simulink model "CRL_MCLV_V2_33EP256MC506_SlidingModeObserver_DualShunt_R2015a"  (R2015a)
settings: Solver=FixedStepDiscrete  StartTime=0.0  StopTime=10.0  FixedStep=.00005  RelTol=1e-3
PreLoadFcn:
  | UserParams;
values from neighbouring files (symbols this model uses):
  DELTA_STARTUP_RAMP = round( (MINSPEEDINRPM*POLEPAIRS*LOOPTIMEINSEC*LOOPTIMEINSEC*65536*65536/(60*OPENLOOPTIMEINSEC)) )    [UserParams.m]
  TS = LOOPTIMEINSEC    (= 5e-05)    [UserParams.m]
undefined symbols (not defined in the file or in its folder): A4, B15, B9, C5, C6, D8, F0, F1, Max, ms, P20, P41, P47, P53, P54, P96, P97, Pin, PWMmax, Resol, us
libraries: MCHP_Blockset x18, simulink x12
(part 1 of 2)
settings Model: Creator=M91449  LastModifiedBy=Lubin Kerhuel
settings DataIOCC: SaveFormat=Dataset
settings OptimizationCC: InlineParams=on  InlineInvariantSignals=on  OptimizeModelRefInitCode=on  LifeSpan=1
settings HardwareCC: ProdBitPerInt=16  ProdBitPerPointer=16  ProdLargestAtomicInteger=Integer  ProdIntDivRoundTo=Zero  ProdEndianess=LittleEndian  ProdWordSize=16  ProdHWDeviceType=Generic->Custom
settings ModelReferenceCC: ModelReferenceNumInstancesAllowed=Single
settings RTWCC: SystemTargetFile=MCHP_dsPIC_stf.tlc  TemplateMakefile=MCHP_dsPIC.tmf  Description=Microchip Embedded Target PIC24 dsPIC30 dsPIC33 (real-time)  GenerateReport=on  IncludeHyperlinkInReport=on  LaunchReport=on  GenerateTraceInfo=on  GenerateTraceReport=on  GenerateTraceReportSl=on  GenerateTraceReportSf=on  GenerateTraceReportEml=on  GenerateWebview=on  GenerateCodeMetricsReport=on  GenerateCodeReplacementReport=on
settings CodeAppCC: IgnoreCustomStorageClasses=off  MaxIdLength=255
settings STFCustomTargetCC: TargetLibSuffix=_lib.a  CodeReplacementLibrary=Microchip Code Replacement Library for dsPIC  GenerateSampleERTMain=off  IncludeMdlTerminateFcn=off  CombineOutputUpdateFcns=on  SuppressErrorStatus=on  SupportContinuousTime=off  SupportNonInlinedSFcns=on  SupportVariableSizeSignals=off  SystemTargetFile=MCHP_dsPIC_stf.tlc
settings ERTTargetCC: TargetLibSuffix=_lib.a  CodeReplacementLibrary=Microchip Code Replacement Library for dsPIC  GenerateSampleERTMain=off  IncludeMdlTerminateFcn=off  SuppressErrorStatus=on  SupportContinuousTime=off  SupportNonInlinedSFcns=on  SupportVariableSizeSignals=off  ERTSrcFileBannerTemplate=MCHP_dsPIC_code_template.cgt  ERTHdrFileBannerTemplate=MCHP_dsPIC_code_template.cgt  ERTDataSrcFileTemplate=MCHP_dsPIC_code_template.cgt  ERTDataHdrFileTemplate=MCHP_dsPIC_code_template.cgt  ERTCustomFileTemplate=MCHP_main.tlc

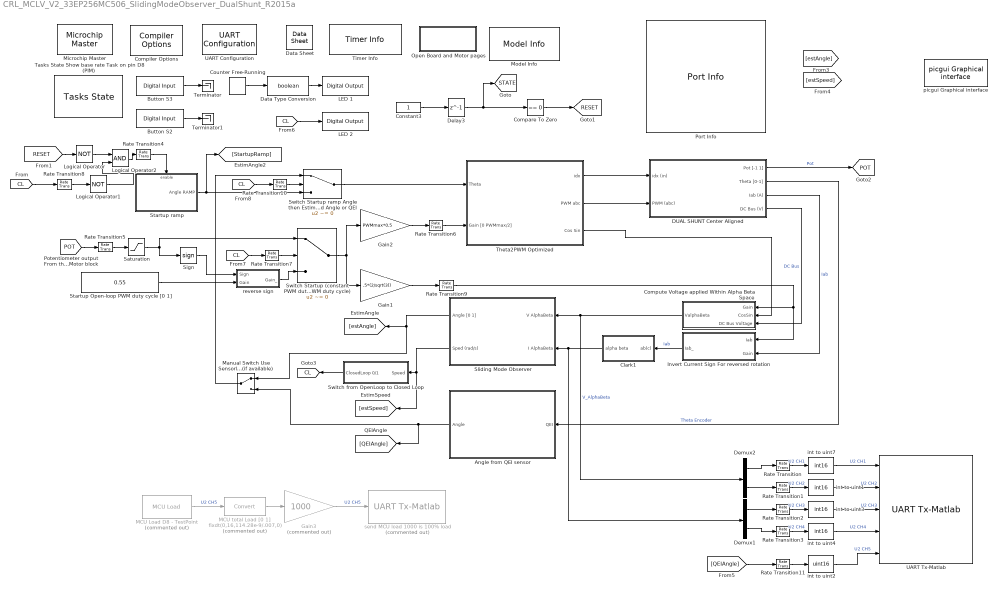
== system CRL_MCLV_V2_33EP256MC506_SlidingModeObserver_DualShunt_R2015a ==
  Angle from QEI sensor : Subsystem
  Button S2 : MCHP_Blockset/Digital IO/Digital Input  PORT=Dynamic Options  PORT_TXT="G   [ 6 : 9 ]"  PIN=7  PACK=off  SIMULTANEOUS=off  ORDERING=None  SampleTime=.1  MCHP_PORT={Digital In}{DIN}2:0:G7;  MCHP_MASTERLINK=CRL_MCLV_V2_33EP256MC506_SlidingModeObserver_DualShunt_R2015a/Microchip Master
  Button S3 : MCHP_Blockset/Digital IO/Digital Input  PORT=Dynamic Options  PORT_TXT="G   [ 6 : 9 ]"  PIN=6  PACK=off  SIMULTANEOUS=off  ORDERING=None  SampleTime=.1  MCHP_PORT={Digital In}{DIN}2:0:G6;  MCHP_MASTERLINK=CRL_MCLV_V2_33EP256MC506_SlidingModeObserver_DualShunt_R2015a/Microchip Master
  Clark1 : Subsystem
  Compare To Zero : simulink/Logic and Bit Operations/Compare To Zero  relop===  OutDataTypeStr=boolean
  Compiler Options : MCHP_Blockset/System Configuration/Compiler Options  Priority=1  LATEST_CMPLR=on  COMP_LIST=Dynamic Options  COMP_LIST_TXT=xc16 - v1.35  USE_64BIT_DOUBLE=off  MCHP_MULTITHREAD_COMPILATION=on  UseCustom_LinkerScript=off  MCHP_MASTERLINK=CRL_MCLV_V2_33EP256MC506_SlidingModeObserver_DualShunt_R2015a/Microchip Master  OPTIMIZATION_LEVEL=3  MPLAB_LINKLIB=default  MPLAB_LINKLIB1=default  UNROLL_LOOPS=on  OMIT_FRAME_POINTER=off  PROCEDURAL_ABSTRACTION=off  MCONST=in data memory  MDATA=Use only memory below address 8192 (faster)  MSCALAR=Use only memory below address 8192 (faster)  MCODE=is less than 32768 (faster)  HEAP_SIZE=0  OMF=elf  DEBUG_INFO=off  AssemblyListing=off  ProduceHexOutput=on
  Compute Voltage applied Within Alpha Beta Space : Subsystem
  Constant3 : Constant  OutDataTypeStr=uint16  SampleTime=.1
  Counter Free-Running : simulink/Sources/Counter Free-Running  NumBits=1  tsamp=.1
  DUAL SHUNT Center Aligned : Subsystem  VariantControl=(default)
  Data Sheet : MCHP_Blockset/System Info/Data Sheet  DOC_Type=datasheet  DOC_MCHP_Id=33EP256MC506_datasheet  DOC_FilePath=C:\Users\M91449\AppData\Local\Temp\70000657H.pdf  DOC_FileLastCheckTime="[2016              1             28             13             25         44.133]"  cpy_MCHP_Id=33EP256MC506  MCHP_MASTERLINK=CRL_MCLV_V2_33EP256MC506_SlidingModeObserver_DualShunt_R2015a/Microchip Master
      settings: AttributesFormatString=%<cpy_MCHP_Id>
  Data Type Conversion : DataTypeConversion  OutDataTypeStr=boolean
  Delay3 : Delay  DelayLength=1  InitialCondition=0
  Demux1 : Demux  Outputs=2
  Demux2 : Demux  Outputs=2
  Gain1 : Gain  Gain=.5*(2/sqrt(3))  OutDataTypeStr=fixdt(1,16,15)
  Gain2 : Gain  Gain=PWMmax*0.5  OutMin=-PWMmax*0.5  OutMax=PWMmax*0.5  OutDataTypeStr=fixdt(1,16)
  Gain3 : Gain  Commented=on  Gain=1000  OutDataTypeStr=uint16
  Invert Current Sign For reversed rotation : Subsystem
  LED 1 : MCHP_Blockset/Digital IO/Digital Output  PORT=Dynamic Options  PORT_TXT="D   [ 5  6  8 ]"  PIN=6  PACK=off  SIMULTANEOUS=off  READPREVIOUS=off  ORDERING=None  SampleTime=-1  MCHP_MASTERLINK=CRL_MCLV_V2_33EP256MC506_SlidingModeObserver_DualShunt_R2015a/Microchip Master
  LED 2 : MCHP_Blockset/Digital IO/Digital Output  PORT=Dynamic Options  PORT_TXT="D   [ 5  6  8 ]"  PIN=5  PACK=off  SIMULTANEOUS=off  READPREVIOUS=off  ORDERING=None  SampleTime=-1  MCHP_MASTERLINK=CRL_MCLV_V2_33EP256MC506_SlidingModeObserver_DualShunt_R2015a/Microchip Master
  Logical Operator : Logic  Operator=NOT  AllPortsSameDT=off  OutDataTypeStr=boolean
  Logical Operator1 : Logic  Operator=NOT  AllPortsSameDT=off  OutDataTypeStr=boolean
  Logical Operator2 : Logic  AllPortsSameDT=off  OutDataTypeStr=boolean
  MCU Load D8 - TestPoint : MCHP_Blockset/Profiling/MCU Load  Commented=on  MCULoadPin=Dynamic Options  MCULoadPin_TXT=None  MCULoadMeasure=on  TIMER_Resolution=Dynamic Options  TIMER_Resolution_TXT="Resol: 0.1143(us)  -  Max: 7.49(ms)"  MCHP_TIMER_REQUEST={MCU_Load}{MCU_Load}21:5:0:0:[]:524288;  MCHP_TIMER_RESULT=[1 65535 ]  MCHP_MASTERLINK=CRL_MCLV_V2_33EP256MC506_SlidingModeObserver_DualShunt_R2015a/Microchip Master  MCHP_COMPILED_INFO="CompiledSampleTime= [0.0070000000000000001   0 ];CompiledInportDataTypes=[ ];CompiledInportDataWidth=[];"  Info="Timer 1:  Resol: 114.2857143(ns)  -  Max: 7.48983(ms)"  SampleTime=.007
  MCU total Load [0 1] : DataTypeConversion  Commented=on  OutDataTypeStr=fixdt(0,16,114.28e-9/.007,0)  ConvertRealWorld=Stored Integer (SI)
  Manual Switch Use Sensorless Estimation or QEI (if available) : ManualSwitch
  Microchip Master : MCHP_Blockset/System Configuration/Microchip Master  Priority=1  PICREF=33EP256MC506  TIMESTEP_REF=ADC  BUSYFLAG=Dynamic Options  BUSYFLAG_TXT=D8 / Pin[42]  PWRTEN=Not used  BOREN=Disable  BODENV=2.7V  BORV=Not used  FPWRT=128ms  DSBOREN=Enable ZPBOR during Deep Sleep Mode  DSLPBOR=Not used  MCLRE=Enabled  SMCLR=MCLR pin generates a normal system Reset  PMDL1WAY=Allow only one reconfiguration  RSTPRI=Device will obtain reset instruction from Primary flash  TEMP=Not used  SOSCSRC=Not used  SOSCSEL=Not used  IOL1WAY=Allow only one reconfiguration  ALTVREF=Not used  DISUVREG=Not used  DSSWEN=Not used  LPCFG=Not used  RTCBAT=Not used  VBTBOR=Not used  WUTSEL=Not used  POWERSAVE=off  FNOSC=Primary Oscillator (XT; HS; EC)  FPR=ECIO w/ PLL 16x  FOSFPR=HS3 w/PLL 16x  FOS=Primary Oscillator  FRANGE=High Range  OSCILLATOR_SELECT=Crystal / Ceramic resonator  OSCILLATOR_SELECT_spd=Crystal / Ceramic resonator  QUARTZ=8e6  QUARTZ_spd=8e6  POSCGAIN=2x gain setting  POSCBOOST=Boost the kick start of the oscillator  SOSCGAIN=2x gain setting  SOSCBOOST=Boost the kick start of the oscillator  ACTIV_PLL=on  ACTIV_PLL_spd=on  MIPS_DESIRED=70e6  MIPS_DESIRED_spd=70e6  FPLLMUL=Not used  FPLLIDIV=8x Divider  POSCFREQ=Not used  POSCMD=XT Crystal Oscillator Mode  POSCMOD=Primary Oscillator Disabled  MIPS=70 * 1e6  ACLKCON=Optimized for PWM resolution & ADC conversion speed  FPLLODIV=32x Divider  PLLKEN=Clock switch to PLL source will wait until the PLL lock signal is valid.  FCKSM=Both Clock switching and Fail-safe Clock Monitor are enabled  FCKSMEN=Sw Disabled; Mon Disabled  IESO=Start up with FRC; then switch  DSWDTPS=1:2^36  FWDTEN=Disable  FWDTWINSZ=Window size is 25%  FWPSA=1:512  FWPSA0=1:128  FWPSB=1:16  WDT=Disable  WDTPOST=1:32768  WDTPRE=1:128  WDTPS=1:32768  WINDIS=Watchdog Timer in Non-Window mode  WWDTEN=Non-Window mode  DSWDTEN=Enable DSWDT during Deep Sleep Mode  DSWDTOSC=Select LPRC as DSWDT Reference clock  FPBDIV=Not used  FSOSCEN=Enable SOSC  LPRCSEL=Not used  OSCIOFCN=Not used  OSCIOFNC=general purpose digital I/O pin  LVRCFG=Not used  PLL_96MHZ=Not used  PLL96MHZ=Not used  PLLDIV=Not used  WDTCLK=Not used  WDTCMX=Not used  WDTWIN=WDT Window is 25% of WDT period  APL=Aux Flash Code protect is disabled  APLK=Aux Flash Write Protection or Code Protection is Enabled  AWRP=Auxiliary program memory is not write-protected  BSS=No Boot program Flash segment  BWP=Not used  BWRP=Boot Segment may be written  CP=Protection Disabled  EBS=No Boot EEPROM  ESS=No Segment Data EEPROM  GCP=General Segment Code protect is Disabled  GSS=General Segment Code protect is Disabled  GSS0=Not used  GSSK=General Segment Write Protection or Code Protection is Enabled  GWRP=General Segment may be written  PWP=Not used  RBS=No Boot RAM  RSS=No Secure RAM  SSS=No Secure Segment  SWRP=Secure segment may be written  WPCFG=Not used  WPDIS=Not used  WPEND=Not used  WPFP=Not used  ICESEL=Communicate on PGEC1/PGED1  ICS=Communicate on PGEC2 and PGED2  JTAGEN=Disable  COE=Not used  RES=Not used  DEBUG=Debugger is disabled  BACKBUG=Not used  BKBUG=Not used  ALTI2C=I2C mapped to SDA1/SCL1 pins  ALTI2C1=I2C1 mapped to SDA1/SCL1 pins  ALTI2C2=I2C2 mapped to SDA2/SCL2 pins  ALTQIO=QEA1; QEB1; INDX1 are selected as inputs to QEI1  ALTSS1=SS1A is selected as the I/O pin for SPI1  CMPPOL0=Hysteresis is applied to falling edge  CMPPOL1=Hysteresis is applied to falling edge  FCANIO=Not used  FETHIO=Default Ethernet I/O  FMIIEN=MII Enabled  FSRSSEL=Not used  FUSBIDIO=Controlled by the USB Module  FVBUSONIO=Not used  HPOL=PWM module high side output pins have active-high output polarity  HYST0=45 mV Hysteresis  HYST1=45 mV Hysteresis  I2C1SEL=Not used  LPOL=PWM module low side output pins have active-high output polarity  PWMPIN=PWM module pins controlled by PORT register at device Reset  RTCOSC=Not used  UPLLEN=USB PLL Disabled  UPLLIDIV=Not used  ATMOD8=Not used  ALTPMP=Not used  I2C2SEL=Not used  ALTADREF=Not used  ALTCVREF=Not used  PWMLOCK=PWM registers may be written without key sequence  MCHP_TIMER_RESULT=[ ]  MCHP_PORT={Busy Flag}{Busy}0:1:D8;  MCHP_PLLRegisters="[5    243  16385     -1]"  MCHPVAR=MCHP.fcy.MIPS=70000000;MCHP.fcy.SYSCLK=70000000;MCHP.fcy.ADC=70000000;MCHP.fcy.Comparator=70000000;MCHP.fcy.I2C=70000000;MCHP.fcy.SPI=70000000;MCHP.fcy.UART=70000000;MCHP.fcy.Timers=70000000;MCHP.fcy.OC=70000000;MCHP.fcy.IC=70000000;MCHP.fcy.Ports=70000000;MCHP.fcy.QEI=70000000;MCHP.PowerSave=0;MCHP.TimeStepFactor=-20000;MCHP.TimeStep_Timer=-1;MCHP.NTIMERS=5;MCHP.id.name='33EP256MC506';MCHP.id.N=reshape([33 256 506],1,3);MCHP.id.L=reshape({ 'EP','MC',''},1,3);MCHP.id.Arch=3;MCHP.periph.PPS.reg_RPINRx=reshape([-1 1 1 -1 -1 -1 1 -1 -1 -1 -1 -1 -1 -1 1 1 1 1 -1 -1 -1 -1 -1 -1 1 1 -1 -1 1 1 1 1 -1 -1 -1 -1 1 -1 1 -1 -1 -1 -1 -1 1 1 1 -1 -1 -1 -1 -1 1 -1 -1 -1 -1 -1 -1 -1 -1 -1 -1 -1 -1 -1 -1 -1 -1 -1 -1 -1 -1 -1 -1 1 -1 1 1 1],1,80);MCHP.PPS.dsPIC.RP=reshape([-1 -1 -1 -1 -1 -1 -1 -1 -1 -1 -1 -1 -1 -1 -1 -1 -1 -1 -1 -1 4 -1 -1 -1 -1 -1 -1 -1 -1 -1 -1 -1 -1 -1 -1 19 20 21 22 23 24 25 26 27 -1 -1 -1 -1 -1 -1 -1 -1 -1 -1 38 39 40 41 -1 -1 -1 -1 -1 -1 -1 -1 -1 -1 -1 -1 -1 -1 -1 -1 -1 -1 -1 -1 -1 -1 -1 -1 -1 -1 -1 -1 -1 -1 -1 -1 -1 -1 -1 -1 -1 -1 -1 81 -1 -1 -1 -1 -1 -1 -1 -1 -1 -1 -1 -1 -1 -1 -1 -1 -1 -1 -1 -1 102 -1 104],1,121);MCHP.PPS.dsPIC.RPI=reshape([-1 -1 -1 -1 -1 -1 -1 -1 -1 -1 -1 -1 -1 -1 -1 -1 -1 -1 -1 -1 -1 -1 -1 -1 8 9 -1 11 12 -1 -1 -1 16 17 18 -1 -1 -1 -1 -1 -1 -1 -1 -1 28 29 30 31 -1 -1 -1 35 36 37 -1 -1 -1 -1 42 -1 -1 -1 -1 -1 -1 -1 -1 -1 -1 -1 -1 -1 -1 -1 -1 -1 -1 -1 -1 -1 -1 -1 -1 -1 -1 -1 -1 -1 -1 -1 -1 -1 -1 -1 78 79 80 -1 -1 -1 -1 -1 -1 -1 -1 -1 -1 -1 -1 -1 -1 -1 -1 -1 -1 -1 -1 -1 -1 103 -1 105],1,122);MCHP.PPS.dsPIC.RPINR_list=reshape({ '1','INT1','INT2','INT3','INT4','T1CK','T2CK','T3CK','T4CK','T5CK','T6CK','T7CK','T8CK','T9CK','IC1','IC2','IC3','IC4','IC5','IC6','IC7','IC8','OCFA','OCFB','FLT1','FLT2','FLT3','FLT4','QEA1','QEB1','INDX1','HOME1','QEA2','QEB2','INDX2','HOME2','U1RX','U1CTS','U2RX','U2CTS','SDI1','SCK1_in','SS1_in','44','SDI2','SCK2_in','SS2_in','48','CSDIR','CSCK','COFS','52','C1RX','C2RX','U3RX','U3CTS','U4RX','U4CTS','SDI3','SCK3_in','SS3_in','62','SDI4','SCK4_in','SS4_in','66','IC9','IC10','IC11','IC12','IC13','IC14','IC15','IC16','OCFC','SYNCI1','SYNCI2','DTCMP1','DTCMP2','DTCMP3','DTCMP4','DTCMP5','DTCMP6','DTCMP7','FLT5','FLT6','FLT7','FLT8','89','SENT1','SENT2','92'},1,92);MCHP.PPS.dsPIC.RPOR_list=reshape({ '1','U1TX','U1RTS','U2TX','U2RTS','SDO1','SCK1_out','SS1_out','SDO2','SCK2_out','SS2_out','CSDO','CSCK','COFS','C1TX','C2TX','OC1','OC2','OC3','OC4','OC5','OC6','OC7','OC8','C1OUT','C2OUT','C3OUT','U3TX','U3RTS','U4TX','U4RTS','SDO3','SCK3_out','SS3_out','SDO4','SCK4_out','SS4_out','OC9','OC10','OC11','OC12','OC13','OC14','OC15','OC16','SYNCO1','SYNCO2','QEI1CCMP','QEI2CCMP','REFCLK','C4OUT','C5OUT','52','53','54','55','56','SENT1','SENT2'},1,59);MCHP.PPS.map_RPnR_RPORx=reshape([20 35 36 37 38 39 40 41 42 43 54 55 56 57 -1 97 -1 118 120],1,19);MCHP.Rx=reshape([13 15 21 -1 -1 58 -1 -1 -1 -1 -1 14 16 22 -1 -1 59 -1 -1 -1 -1 -1 -1 17 23 -1 -1 -1 -1 -1 -1 -1 -1 -1 18 35 -1 -1 -1 -1 -1 -1 -1 -1 33 32 36 -1 -1 -1 -1 -1 -1 -1 -1 -1 43 37 53 -1 -1 -1 -1 -1 -1 -1 -1 44 50 54 -1 -1 4 -1 -1 -1 -1 1 46 51 -1 -1 -1 5 -1 -1 -1 -1 31 48 52 42 -1 -1 6 -1 -1 -1 -1 34 49 55 -1 -1 -1 8 -1 -1 -1 -1 64 60 45 -1 -1 -1 -1 -1 -1 -1 -1 12 61 24 -1 -1 -1 -1 -1 -1 -1 -1 11 62 39 -1 27 -1 -1 -1 -1 -1 -1 -1 63 47 -1 28 -1 -1 -1 -1 -1 -1 -1 2 -1 -1 29 -1 -1 -1 -1 -1 -1 -1 3 40 -1 30 -1 -1 -1 -1 -1 -1],11,16);MCHP.ADC.ANtype=reshape([3 0],1,2);MCHP.ADC.ADCONx=reshape([47103 59391 40959 263 0 0],1,6);MCHP.ADC.ADCHS_0=reshape([40863 1799],1,2);MCHP.ADC.Flags=reshape([1 0],1,2);MCHP.ADC.Buffer=reshape([16 -1],1,2);MCHP.ADC.port=reshape([0 1 16 17 18 19 32 33 34 11 12 43 76 77 78 79 -1 -1 -1 -1 -1 -1 -1 -1 -1 -1 -1 -1 -1 -1 -1 -1 -1 -1 -1 -1 -1 -1 -1 -1 -1 -1 -1 -1 -1 -1 -1 -1 -1 -1 -1 -1 -1 -1 -1 -1 -1],1,57);MCHP.ADC.port_ALT=reshape([-1 -1 -1 -1],1,4);MCHP.ADC.port_VrefP=17;MCHP.ADC.port_VrefM=16;MCHP.ADC.port_AVdd=-1;MCHP.ADC.port_AVss=-1;MCHP.ADC.ADCDATA=reshape([0 0 0 0 0 0 0 0 0 0 0 0 0 0 0 0 0 0 0 0 0 0 0 0 0 0 0 0 0 0 0 0 0 0 0 0 0 0 0 0 0 0 0 0 0 0 0 0 0 0 0 0 0 0 0 0 0],1,57);MCHP.memory.RAM=32768;MCHP.memory.RAM_XBegin=4096;MCHP.memory.RAM_YBegin=20480;MCHP.memory.RAM_dma=reshape([-1 -1],1,2);MCHP.memory.FLASH_ECC=0;MCHP.DMA.Num=4;MCHP.DMA.CNTmax=16383;MCHP.QEI.QEICONx=reshape([49023 -1 -1 -1 -1 -1],1,6);MCHP.QEI.QEItype=1;MCHP.QEI.Port_QEI_INDX=reshape([-1 -1],1,2);MCHP.QEI.Port_QEI_QEA=reshape([-1 -1],1,2);MCHP.QEI.Port_QEI_QEB=reshape([-1 -1],1,2);MCHP.QEI.Port_QEI_UPDN=reshape([-1 -1],1,2);MCHP.INT.Port=reshape([23 32767 32767 -1 -1],1,5);MCHP.PWM_HS.Flags=reshape([3 1 0],1,3);MCHP.PWM.port_FLT=reshape([-1 -1 -1 34 43 -1 -1 -1 -1 -1 -1 -1 -1 -1 -1 -1 -1 -1 -1 -1 -1 -1 -1 -1 -1 -1 -1 -1 -1 -1 -1 -1 20],1,33);MCHP.PWM.PWMRef=-1;MCHP.PWM.Flag=0;MCHP.PWM.Port_PWM_l=reshape([31 -1 29 -1 27 -1 -1 -1 -1 -1 -1 -1 -1 -1 -1 -1 -1 -1 -1 -1 -1 -1 -1 -1],2,12);MCHP.PWM.Port_PWM_h=reshape([30 -1 28 -1 26 -1 -1 -1 -1 -1 -1 -1 -1 -1 -1 -1 -1 -1 -1 -1 -1 -1 -1 -1],2,12);MCHP.IC.Port=reshape([32767 32767 32767 32767 0 0 0 0 0 0 0 0 0 0 0 0],1,16);MCHP.IC.type=1;MCHP.OC.Port=reshape([32767 32767 32767 32767 0 0 0 0 0 0 0 0 0 0 0 0],1,16);MCHP.OC.type=1;MCHP.CN.Port=reshape([-1 -1 -1 -1 -1 -1 -1 -1 -1 -1 -1 -1 -1 -1 -1 -1 -1 -1 -1 -1 -1 -1 -1 -1 -1 -1 -1 -1 -1 -1 -1 -1 -1 -1 -1 -1 -1 -1 -1 -1 -1 -1 -1 -1 -1 -1 -1 -1 -1 -1 -1 -1 -1 -1 -1 -1 -1 -1 -1 -1 -1 -1 -1 -1 -1 -1 -1 -1 -1 -1 -1 -1 -1 -1 -1 -1 -1 -1 -1 -1 -1 -1 -1 -1 -1],1,85);MCHP.CN.PullUp=reshape([8083 65535 49151 352 61440 3 960 0 0 0 0],1,11);MCHP.CN.type=1;MCHP.CN.Flag_PullDown=1;MCHP.SPI.Refs=reshape([1 2 0 0 0 0],1,6);MCHP.SPI.SPIxCON1=8191;MCHP.SPI.SPIxCON2=57347;MCHP.SPI.Port_SDI=reshape([9 -1 -1 -1 -1 -1],1,6);MCHP.SPI.Port_SDO=reshape([4 -1 -1 -1 -1 -1],1,6);MCHP.SPI.Port_SCK=reshape([35 -1 -1 -1 -1 -1],1,6);MCHP.SPI.Port_SS=reshape([16 -1 -1 -1 -1 -1],1,6);MCHP.I2C.Refs=reshape([1 2 0 0 0],1,5);MCHP.I2C.I2CxCON=49151;MCHP.I2C.NewRegName=1;MCHP.I2C.Port_SDA=reshape([36 8 -1 -1 -1],1,5);MCHP.I2C.Port_SCL=reshape([37 20 -1 -1 -1],1,5);MCHP.I2C.Port_ASDA=reshape([25 21 -1 -1 -1],1,5);MCHP.I2C.Port_ASCL=reshape([24 22 -1 -1 -1],1,5);MCHP.I2C.Fuse_Port_SCL_SDA=reshape([3 1 4 1 -1 -1 -1 -1 -1 -1],2,5);MCHP.I2C.Fuse_Port_ASCL_ASDA=reshape([3 2 4 2 -1 -1 -1 -1 -1 -1],2,5);MCHP.PGA.Port_PGA1P=reshape([-1 -1 -1 -1],1,4);MCHP.PGA.Port_PGA1N=reshape([-1 -1 -1 -1],1,4);MCHP.PGA.Port_PGA2P=reshape([-1 -1 -1 -1],1,4);MCHP.PGA.Port_PGA2N=reshape([-1 -1 -1 -1],1,4);MCHP.PGA.Num=0;MCHP.HS_AnalogComparator.Port_CMP1=reshape([-1 -1 -1 -1],1,4);MCHP.HS_AnalogComparator.Port_CMP2=reshape([-1 -1 -1 -1],1,4);MCHP.HS_AnalogComparator.Port_CMP3=reshape([-1 -1 -1 -1],1,4);MCHP.HS_AnalogComparator.Port_CMP4=reshape([-1 -1 -1 -1],1,4);MCHP.HS_AnalogComparator.PORT_EXTREFx=reshape([-1 -1],1,2);MCHP.HS_AnalogComparator.Port_DACOUTx=reshape([-1 -1],1,2);MCHP.HS_AnalogComparator.Num=0;MCHP.Comp.Port_CVrefin=-1;MCHP.Comp.Port_CVref=-1;MCHP.Comp.Port_CVref1O=24;MCHP.Comp.Port_CVref2O=4;MCHP.Comp.Port_CxOUT=reshape([32767 32767 32767 32767 -1],1,5);MCHP.Comp.Port_OAxOUT=reshape([17 0 32 -1 -1],1,5);MCHP.Comp.Port_CxINP=reshape([18 1 34 32 -1],1,5);MCHP.Comp.Port_CxINM=reshape([19 43 -1 -1 16 76 -1 -1 33 77 -1 -1 33 -1 -1 -1 -1 -1 -1 -1],4,5);MCHP.Comp.nComp=reshape([4 0 0],1,3);MCHP.Comp.OpAmp=7;MCHP.Comp.CVRCON=reshape([17663 0],1,2);MCHP.CDAC.Port_DACx=reshape([-1 -1 -1],1,3);MCHP.CDAC.nCDAC=0;MCHP.UART.port_Rx=reshape([32767 32767 -1 -1 -1 -1],1,6);MCHP.UART.port_Tx=reshape([32767 32767 -1 -1 -1 -1],1,6);MCHP.UART.port_ARx=reshape([-1 -1],1,2);MCHP.UART.port_ATx=reshape([-1 -1],1,2);MCHP.UART.port_RTS=reshape([34 76 -1 -1 -1 -1],1,6);MCHP.UART.port_CTS=reshape([43 77 -1 -1 -1 -1],1,6);MCHP.UART.reg_UxMODE=reshape([48127 48127 -1 -1 -1 -1],1,6);MCHP.UART.reg_UxSTA=reshape([61439 61439 -1 -1 -1 -1],1,6);MCHP.modsrc.DOS_00794=1;MCHP.modsrc.DOS_00931=1;MCHP.modsrc.DOS_00932=1;MCHP.modsrc.DOS_00942=1;MCHP.modsrc.DOS_00938=1;MCHP.modsrc.DOS_00996=1;MCHP.modsrc.DOS_00997=1;MCHP.modsrc.DOS_00998=1;MCHP.modsrc.DOS_00209=0;MCHP.modsrc.DOS_01555_adc=0;MCHP.modsrc.DOS_01293=1;MCHP.modsrc.DOS_00828=0;MCHP.modsrc.DOS_01116=1;MCHP.modsrc.DOS_01017_RPORx=1;MCHP.modsrc.DOS_01017_RPINRx=1;MCHP.modsrc.DOS_01555_nvm_tsmc18_v2_16bit=0;MCHP.modsrc.DOS_00804=1;MCHP.modsrc.DOS_00826=1;MCHP.modsrc.DOS_01555_TLAK_PMDx=0;MCHP.modsrc.DOS_01555_TLAK_INT_=0;MCHP.modsrc.DOS_00933=1;MCHP.modsrc.DOS_01555=0;MCHP.modsrc.DOS_01555_ptg=0;MCHP.modsrc.DOS_00929=1;MCHP.modsrc.DOS_00958=1;MCHP.modsrc.DOS_01117_PORTx=1;MCHP.modsrc.DOS_00999=0;MCHP.modsrc.DOS_01198=1;MCHP.modsrc.DOS_01041=1;MCHP.modsrc.DOS_00892=1;MCHP.modsrc.DOS_01287_TLAC_PMDx=1;MCHP.modsrc.DOS_01287_TLAC_INT_=1;MCHP.modsrc.DOS_01424=1;MCHP.modsrc.DOS_01332=1;MCHP.modsrc.DOS_01441_i2c_upb_v1_16bit_TLAH=0;MCHP.modsrc.DOS_01482=0;MCHP.modsrc.DOS_02508c11=0;MCHP.modsrc.DOS_01468_PMBA_current_source=0;MCHP.modsrc.DOS_02291_PGA=0;MCHP.modsrc.DOS_01467_Comparator=0;MCHP.modsrc.DOS_01498_TLAY=0;MCHP.modsrc.DOS_02316_nvm_ctrl_v1_16bit=0;MCHP.modsrc.DOS_00993_PLL_120MHz=0;MCHP.modsrc.DOS_01577_cla_clc_upb_v1=0;MCHP.modsrc.DOS_01332_ptg_pc_v1=0;MCHP.modsrc.DOS_00958_pwm_TLAY=0;MCHP.modsrc.TLAY_IOPorts=0;MCHP.modsrc.DOS_00929q=0;MCHP.modsrc.DOS_02415_spi_v5=0;MCHP.modsrc.DOS_RPINRx_16bit_2=0;MCHP.modsrc.DOS_01497_TLAH_PMDx=0;MCHP.modsrc.DOS_02550_TLAL_INT=0;MCHP.modsrc.DOS_00958_pwm_TLAH=0;MCHP.modsrc.DOS_01287_TLAH_INT_=0;MCHP.modsrc.DOS_01113=0;MCHP.modsrc.DOS_01017_PMDx=0;MCHP.modsrc.DOS_00927=0;MCHP.modsrc.DOS_01080=0;MCHP.modsrc.DOS_00794_cpu_16bit_v3=0;MCHP.modsrc.DOS_02359a_sent_j2716_upb_v1=0;MCHP.modsrc.DOS_01520_wdt_dmt_upb_v1_16bit=0;MCHP.modsrc.DOS_02192_TLCD_PMDx=0;MCHP.modsrc.DOS_02192_TLCD_INT_=0;MCHP.modsrc.DOS_02192_cmp=0;MCHP.modsrc.DOS_00958_pwm_TLCD=0;MCHP.modsrc.DOS_02192_PORTx_TLCD=0;MCHP.modsrc.DOS_00936=0;MCHP.modsrc.DOS_00995=0;MCHP.modsrc.DOS_00546=0;MCHP.modsrc.DOS_00474=0;MCHP.modsrc.DOS_02481_WACJ_Config=0;MCHP.modsrc.DOS_02569_pfm_cache_ocp_v1=0;MCHP.modsrc.DOS_02819_pfm_ctrl_32bit_upb_v2=0;MCHP.modsrc.DOS_02674_wdt_upb_v1_32bit=0;MCHP.modsrc.DOS_01520_wdt_dmt_upb_v1=0;MCHP.modsrc.DOS_02869_icd_jtag_bvci_upb_v2=0;MCHP.modsrc.DOS_02823_WACJ_clk_cru_upb_v2=0;MCHP.modsrc.DOS_01423_RPINRx=0;MCHP.modsrc.DOS_02481_RPORx=0;MCHP.modsrc.DOS_02511_pwr_sib_upb_v1_32bit=0;MCHP.modsrc.DOS_02481_WACJ_int_evic_v3=0;MCHP.modsrc.DOS_01500_dma_bvci_v2=0;MCHP.modsrc.DOS_02141_tmr_classa_pb_v2=0;MCHP.modsrc.DOS_02815_tmr_classb_upb_v1=0;MCHP.modsrc.DOS_00740_icap_pb_v1=0;MCHP.modsrc.DOS_00749_ocmp_pb_v1=0;MCHP.modsrc.DOS_01441_i2c_upb_v1_32bit=0;MCHP.modsrc.DOS_01329_spi_pb_v2=0;MCHP.modsrc.DOS_02478_uart_irda_upb_v1_32bit=0;MCHP.modsrc.DOS_02514_dfm_strl_sst_upb_v1=0;MCHP.modsrc.DOS_01427_cmp_control_upb_v1_32bit=0;MCHP.modsrc.DOS_01445_dac_nbit__control_upb_v1_32bit=0;MCHP.modsrc.DOS_01461_afe_ctmu_con_upb_v1=0;MCHP.modsrc.DOS_02472_ppi_pmp16_upb_v1=0;MCHP.modsrc.DOS_02467_gpio_ports_upb_v1=0;MCHP.modsrc.DOS_02508_adc_sar_ctrl_upb_v1_PIC32MK=0;MCHP.modsrc.DOS_02813a_usb_otgcore_pb_v3=0;MCHP.modsrc.DOS_01261_tmr_rtcc_pb_v2=0;MCHP.modsrc.DOS_01475_lpwr_deep_sleep_ctrl_v2=0;MCHP.modsrc.DOS_EIP_00136_ssx_v1=0;MCHP.modsrc.DOS_01152_can_bvci_v1=0;MCHP.modsrc.DOS_02481_WACN_Config=0;MCHP.modsrc.DOS_02823_WACN_clk_cru_upb_v2=0;MCHP.modsrc.DOS_02481_WACN_int_evic_v3=0;MCHP.modsrc.DOS_03554_cmp_control_upb_v2_32bit=0;MCHP.modsrc.DOS_01577_cla_clc_upb_v1_32bit=0;MCHP.modsrc.DOS_03247_can_fd_upb_v2=0;MCHP.modsrc.DOS_02481_WACK_MC_Config=0;MCHP.modsrc.DOS_03247_can_fd_upb_v2_pic32mk=0;MCHP.modsrc.DOS_02481_WACJ_MC_Config=0;MCHP.modsrc.DOS_02481_WACJ_MC_int_evic_v3=0;MCHP.modsrc.DOS_01477_pwm_mc_upb_v1=0;MCHP.modsrc.DOS_01459_ptg_pc_upb_v1_SIC=0;MCHP.modsrc.DOS_01494_qei_32b_upb_v1=0;MCHP.modsrc.DOS_02481_WACN_MC_Config=0;MCHP.modsrc.DOS_02481_WACN_MC_int_evic_v3=0;MCHP.modsrc.DOS_02787_WACD_Config=0;MCHP.modsrc.DOS_00800_dac_4bit_ctrl_pb_v1=0;MCHP.modsrc.DOS_01539_icd_jtag_pb_v2=0;MCHP.modsrc.DOS_02823_clk_cru_upb_v2=0;MCHP.modsrc.DOS_01423_RPORx=0;MCHP.modsrc.DOS_02907_WACD_int_evic_v3=0;MCHP.modsrc.DOS_00734_uart_irda_pb_v1=0;MCHP.modsrc.DOS_00687_tmr_classa_pb_v1=0;MCHP.modsrc.DOS_00745_tmr_classb_pb_v1=0;MCHP.modsrc.DOS_02508_adc_sar_ctrl_upb_v1=0;MCHP.modsrc.DOS_00866_cmp_control_pb_v2=0;MCHP.modsrc.DOS_01114_eth_bvci_v1=0;MCHP.modsrc.DOS_02831_usb_clk_rst_v2=0;MCHP.modsrc.DOS_01643_pfm_cache_ahb_v2=0;MCHP.modsrc.DOS_EIP_00206r5_sqi_v2=0;MCHP.modsrc.DOS_EIP_00124_usb_hs_otgcore_v1=0;MCHP.modsrc.DOS_EIP_00218_math_rng_ahbs_v2=0;MCHP.modsrc.DOS_EIP_00109_ebi_v1=0;MCHP.modsrc.DOS_EIP_00158_crypto_v1=0;MCHP.clock.PBxDIV=-1;  MCHP_CRC=5766771  BTMODE=Not used  RES1=Not used  PLLSS=Not used  RES2=Not used  ALTCMPI=Not used  BOREN1=Not used  ALTRB6=Not used  RETCFG=Not used  DFMCY=Not used  BSS2=No Boot Segment  BSEN=No Boot Segment  CWRP=Configuration Segment may be written  CSS=No Protection (other than CWRP)  AIVTDIS=Disable Alternate Vector Table  BSLIM=Not used  WDTEN=Disable  BTSWP=BOOTSWP instruction is disabled  DBCC=No Cross Connection between DAC outputs  CTXT1=Not Assigned  CTXT2=Not Assigned  SEQNUM=Not used  nSEQNUM=Not used  BOREN0=Enabled  DMTIVT=Not used  DMTCNT=2^31 (2147483648)  DMTEN=Dead Man Timer is Disabled and can be enabled by software  ON=Not used  USERID=Not used  RESERVED1=Not used  PGL1WAY=Allow only one reconfiguration  FPLLRNG=34-68 MHz Input  FPLLICLK=FRC is input to the System PLL  FPLLMULT=PLL Multiply by 128  UPLLFSEL=USB PLL input is 24 MHz  DMTINTV=Window/Interval value is 127/128 counter value  WDTSPGM=WDT stops during Flash programming  FDMTEN=Deadman Timer is disabled  TRCEN=Trace features in the CPU are enabled  BOOTISA=Boot code and Exception code is MIPS32  FECCCON=ECC and Dynamic ECC are disabled (ECCCON bits are writable)  EXTDDRSIZE=Not used  FSLEEP=Flash is powered down when the device is in Sleep mode  DBGPER=Allow CPU access to all permission regions  EJTAGBEN=Normal EJTAG functionality  TSEQ=Not used  CSEQ=Not used
  Model Info : simulink/Model-Wide Utilities/Model Info  Frame=on  DisplayStringWithTags=|  HorizontalTextAlignment=Left  LeftAlignmentValue=0.02  SourceBlockDiagram=CRL_MCLV_V2_33EP256MC506_SlidingModeObserver_DualShunt_R2015a  TagMaxNumber=20
      | Short hust motor with:
      | M1 - Black
      | M2 - Red
      | M3 - White
  Open Board and Motor pages : Subsystem
      settings: OpenFcn=|
      | web('www.microchip.com/DevelopmentTools/ProductDetails.aspx?PartNO=DM330021-2','-browser');
      | pause(1);
      | web('http://www.microchipdirect.com/productsearch.aspx?keywords=AC300020','-browser');
      | pause(1);
      | web('www.microchipdirect.com/ProductSearch.aspx?keywords=AC300022','-browser');
      mask Display: disp('Open tools\nWebpage');
  Port Info : MCHP_Blockset/System Info/Port Info  MCHP_MASTERLINK=CRL_MCLV_V2_33EP256MC506_SlidingModeObserver_DualShunt_R2015a/Microchip Master
  Rate Transition{,1..4,6..11} (11 alike) : RateTransition
  Rate Transition5 : RateTransition  OutPortSampleTime=.1
  Saturation : Saturate  UpperLimit=1  LowerLimit=0
  Sign : Signum
  Sliding Mode Observer : Subsystem
  Startup Open-loop PWM duty cycle [0 1] : Constant  Value=0.55  OutDataTypeStr=Inherit: Inherit via back propagation
  Startup ramp : Subsystem
  Switch Startup (constant PWM duty cycle) then Closed Loop (Pot drive PWM duty cycle) : Switch  Criteria=u2 ~= 0  Threshold=250
  Switch Startup ramp Angle then Estimated Angle or QEI : Switch  Criteria=u2 ~= 0  Threshold=250
  Switch from OpenLoop to Closed Loop : Subsystem
  Tasks State Show base rate Task on pin D8 (PIM) : MCHP_Blockset/Profiling/Tasks State  TasksPin=D8  MCHP_PORT={Task D1 Running}{Task D1}15:1:D8;  MCHP_MASTERLINK=CRL_MCLV_V2_33EP256MC506_SlidingModeObserver_DualShunt_R2015a/Microchip Master
  Terminator : Terminator
  Terminator1 : Terminator
  Theta2PWM Optimized : Subsystem  VariantControl=Optimized
  Timer Info : MCHP_Blockset/System Info/Timer Info  MCHP_MASTERLINK=CRL_MCLV_V2_33EP256MC506_SlidingModeObserver_DualShunt_R2015a/Microchip Master
  UART Configuration : MCHP_Blockset/BUS UART/UART Configuration  UART_REF=2  BAUD_Choice=Dynamic Options  BAUD_Choice_TXT="921600         [-0.06%]"  BAUD_Choice_IR=Dynamic Options  BAUD_Choice_IR_TXT=[]  BAUD_Custom=115200  ALT_IO=on  PIN_RX=Dynamic Options  PIN_RX_TXT=C5 / P53 / Pin[37]  PIN_TX=Dynamic Options  PIN_TX_TXT=F1 / P97 / Pin[59]  MCHP_PORT="{UART2  Rx}{U2RX}3:0:P53;{UART2  Tx}{U2TX}3:1:P97;"  MCHP_MASTERLINK=CRL_MCLV_V2_33EP256MC506_SlidingModeObserver_DualShunt_R2015a/Microchip Master  MCHP_COM_ExtPil=off  TX_IMPLEMENTATION=DMA Ping-Pong Mode  TX_IMPLEMENTATION_default=Circular Buffer  TX_INT_PRIORITY=2  TX_INT_WHEN=is empty & last char is sent  TX_INT_WHEN_default=is empty & last char is sent  TX_CIRCULAR_SIZE=32  TX_DMA_CHANNEL="0   (Lowest Priority)"  TX_DMA_SIZE=60  TX_TASK_PROTECTION=Delay tasks (default)  TX_INTERRUPT_PROTECTION=Do not send on conflict (default)  TX_INTERRUPT_PROTECTION_default=Do not send on conflict (default)  RX_IMPLEMENTATION=Simplest (4 bytes internal buffer only)  RX_IMPLEMENTATION_default=Circular Buffer  RX_INT_PRIORITY=1  RX_INT_WHEN=receive 1 character  RX_CIRCULAR_SIZE=32  DuplexMode=Full duplex (default)  PIN_RX_Inv=off  PIN_TX_Inv=off  ParityBit=No parity (default)  StopBit=1 stop bit (default)  IRDA=off  FlowControl=None  PIN_CTS=Dynamic Options  PIN_CTS_TXT=A4 / P20 / Pin[33]  PIN_RTS=Dynamic Options  PIN_RTS_TXT=A4 / P20 / Pin[33]  InitSequence_chkbox=off  BAUD_Choice_InitSeq=Dynamic Options  BAUD_Choice_InitSeq_TXT="110         [-0.00%]"  BAUD_Choice_IR_InitSeq=Dynamic Options  BAUD_Choice_IR_InitSeq_TXT=0  BAUD_Custom_InitSeq=0  InitSequence='Hello World'
  UART Tx-Matlab : MCHP_Blockset/BUS UART/UART Tx-Matlab  UART_REF=2  CHANNELS=[1 2 3 4 5]  AllOrNothing=on  SampleTime=.0002  MCHP_MASTERLINK=CRL_MCLV_V2_33EP256MC506_SlidingModeObserver_DualShunt_R2015a/Microchip Master  MCHP_COMPILED_INFO="CompiledSampleTime= [0.00020000000000000001   0 ];CompiledInportDataTypes=[  4   4   4   4   5 ];CompiledInportDataWidth=[1  1  1  1  1];"
  int to uint{1,3..4,7} (4 alike) : DataTypeConversion  OutDataTypeStr=int16  ConvertRealWorld=Stored Integer (SI)
  int to uint2 : DataTypeConversion  OutDataTypeStr=uint16  ConvertRealWorld=Stored Integer (SI)
  picgui Graphical interface : MCHP_Blockset/BUS UART/picgui Graphical interface  Nothing=0
  reverse sign : Subsystem
  send MCU load 1000 is 100% load : MCHP_Blockset/BUS UART/UART Tx-Matlab  Commented=on  UART_REF=2  CHANNELS=5  AllOrNothing=on  SampleTime=-1  MCHP_MASTERLINK=CRL_MCLV_V2_33EP256MC506_SlidingModeObserver_DualShunt_R2015a/Microchip Master  MCHP_COMPILED_INFO="CompiledSampleTime= [0.0070000000000000001   0 ];CompiledInportDataTypes=[  5 ];CompiledInportDataWidth=[1];"
  tag scope: CL=global, POT=global, RESET=global, STATE=global
  wires:
  Counter Free-Running/1 -> Data Type Conversion/1
  Data Type Conversion/1 -> LED 1/1
  [CL] -> LED 2/1
  Rate Transition/1 -> int to uint7/1  "U2 CH1"
  Rate Transition1/1 -> int to uint1/1  "U2 CH2"
  MCU Load D8 - TestPoint/1 -> MCU total Load [0 1]/1  "U2 CH5"
  Constant3/1 -> Delay3/1
  Delay3/1 -> Compare To Zero/1, [STATE]
  Sliding Mode Observer/2(Sped (rad/s)) -> [estSpeed], Switch from OpenLoop to Closed Loop/1(Speed)
  Switch Startup ramp Angle then Estimated Angle or QEI/1 -> Theta2PWM Optimized/1(Theta)
  Rate Transition2/1 -> int to uint3/1  "U2 CH3"
  Rate Transition3/1 -> int to uint4/1  "U2 CH4"
  Compare To Zero/1 -> [RESET]
  Theta2PWM Optimized/2(PWM abc) -> DUAL SHUNT Center Aligned/2(PWM (abc))
  Startup ramp/1(Angle RAMP) -> [StartupRamp], Switch Startup ramp Angle then Estimated Angle or QEI/3
  [RESET] -> Logical Operator/1
  Rate Transition4/1 -> Startup ramp/Enable
  Theta2PWM Optimized/1(idx) -> DUAL SHUNT Center Aligned/1(idx (in))
  DUAL SHUNT Center Aligned/3(Iab (A)) -> Invert Current Sign For reversed rotation/2(Gain)  "Iab"
  Switch Startup (constant PWM duty cycle) then Closed Loop (Pot drive PWM duty cycle)/1 -> Gain1/1, Gain2/1
  DUAL SHUNT Center Aligned/1(Pot [-1 1]) -> [POT]  "Pot"
  [POT] -> Rate Transition5/1
  Rate Transition5/1 -> Saturation/1
  Saturation/1 -> Sign/1, Switch Startup (constant PWM duty cycle) then Closed Loop (Pot drive PWM duty cycle)/1
  Manual Switch Use Sensorless Estimation or QEI (if available)/1 -> Switch Startup ramp Angle then Estimated Angle or QEI/1
  int to uint3/1 -> UART Tx-Matlab/3  "U2 CH3"
  [CL] -> Rate Transition7/1
  [CL] -> Rate Transition10/1
  Sliding Mode Observer/1(Angle [0 1]) -> Manual Switch Use Sensorless Estimation or QEI (if available)/1, [estAngle]
  Rate Transition9/1 -> Invert Current Sign For reversed rotation/1(Iab), Compute Voltage applied Within Alpha Beta Space/1(Gain)
  Gain2/1 -> Rate Transition6/1
  Rate Transition6/1 -> Theta2PWM Optimized/2(Gain [0 PWMmax/2])
  Gain1/1 -> Rate Transition9/1
  Angle from QEI sensor/1(Angle) -> Manual Switch Use Sensorless Estimation or QEI (if available)/2, [QEIAngle]
  DUAL SHUNT Center Aligned/2(Theta [0-1]) -> Angle from QEI sensor/1(QEI)  "Theta Encoder"
  Invert Current Sign For reversed rotation/1("Iab_ ") -> Clark1/1(ab(c))  "Iab"
  DUAL SHUNT Center Aligned/4(DC Bus (V)) -> Compute Voltage applied Within Alpha Beta Space/3(DC Bus Voltage)  "DC Bus"
  Theta2PWM Optimized/3(Cos Sin) -> Compute Voltage applied Within Alpha Beta Space/2(CosSin)
  Compute Voltage applied Within Alpha Beta Space/1(ValphaBeta) -> Demux2/1, Sliding Mode Observer/1(V AlphaBeta)  "V_AlphaBeta"
  Rate Transition7/1 -> Switch Startup (constant PWM duty cycle) then Closed Loop (Pot drive PWM duty cycle)/2
  Rate Transition10/1 -> Switch Startup ramp Angle then Estimated Angle or QEI/2
  Switch from OpenLoop to Closed Loop/1(ClosedLoop 0/1) -> [CL]
  reverse sign/1(Gain_) -> Switch Startup (constant PWM duty cycle) then Closed Loop (Pot drive PWM duty cycle)/3
  Sign/1 -> reverse sign/1(Sign)
  Startup Open-loop PWM duty cycle [0 1]/1 -> reverse sign/2(Gain)
  int to uint1/1 -> UART Tx-Matlab/2  "U2 CH2"
  int to uint7/1 -> UART Tx-Matlab/1  "U2 CH1"
  int to uint4/1 -> UART Tx-Matlab/4  "U2 CH4"
  MCU total Load [0 1]/1 -> Gain3/1
  Gain3/1 -> send MCU load 1000 is 100% load/1  "U2 CH5"
  Button S3/1 -> Terminator/1
  Button S2/1 -> Terminator1/1
  [CL] -> Rate Transition8/1
  Rate Transition8/1 -> Logical Operator1/1
  Logical Operator/1 -> Logical Operator2/1
  Logical Operator1/1 -> Logical Operator2/2
  Logical Operator2/1 -> Rate Transition4/1
  Clark1/1(alpha beta) -> Demux1/1, Sliding Mode Observer/2(I AlphaBeta)
  Demux2/1 -> Rate Transition/1
  Demux2/2 -> Rate Transition1/1
  Demux1/1 -> Rate Transition2/1
  Demux1/2 -> Rate Transition3/1
  [QEIAngle] -> Rate Transition11/1
  Rate Transition11/1 -> int to uint2/1
  int to uint2/1 -> UART Tx-Matlab/5  "U2 CH5"

== system CRL_MCLV_V2_33EP256MC506_SlidingModeObserver_DualShunt_R2015a/Angle from QEI sensor ==
  QEI : Inport
  Bias : Bias  Bias=0.25
  Gain3 : Gain  Gain=-1  OutDataTypeStr=Inherit: Same as input
  Q0.1 : DataTypeConversion  OutDataTypeStr=fixdt(0,16,16)  ConvertRealWorld=Stored Integer (SI)
  Q0.2 : DataTypeConversion  OutDataTypeStr=int16  ConvertRealWorld=Stored Integer (SI)
  Angle : Outport
  wires:
  Bias/1 -> Angle/1
  Gain3/1 -> Q0.1/1
  Q0.2/1 -> Gain3/1
  Q0.1/1 -> Bias/1
  QEI/1 -> Q0.2/1

== system CRL_MCLV_V2_33EP256MC506_SlidingModeObserver_DualShunt_R2015a/Clark1 ==
  note: Input is a vector of 3 elements, 3rd element is not beeing used
  note: k = 2/3 : invariant Magnitude
  ab(c) : Inport
  Clarke1 : Product  Multiplication=Matrix(*)  OutMin=[-4.4]  OutMax=[4.4]  OutDataTypeStr=fixdt(1,16)  RndMeth=Convergent  SaturateOnIntegerOverflow=on
  Constant Magnitude : Constant  Value=[1 0 ; 1/sqrt(3) 2/sqrt(3) ];  OutDataTypeStr=fixdt(1,16)
  Data Type Conversion : DataTypeConversion  OutMin=-4.4  OutMax=4.4  OutDataTypeStr=fixdt(1,16)  SaturateOnIntegerOverflow=on
  alpha beta : Outport
  wires:
  ab(c)/1 -> Data Type Conversion/1
  Clarke1/1 -> alpha beta/1
  Constant Magnitude/1 -> Clarke1/1
  Data Type Conversion/1 -> Clarke1/2

== system CRL_MCLV_V2_33EP256MC506_SlidingModeObserver_DualShunt_R2015a/Compute Voltage applied Within Alpha Beta Space ==
  Gain : Inport
  CosSin : Inport  Port=2
  DC Bus Voltage : Inport  Port=3
  Abs : Abs  SaturateOnIntegerOverflow=on
  Delay : Delay  InitialCondition=0
  Product1 : Product  OutDataTypeStr=Inherit: Same as first input
  Product3 : Product  OutMin=[-24]  OutMax=[24]  OutDataTypeStr=fixdt(1,16)
  ValphaBeta : Outport
  wires:
  Abs/1 -> Product1/2
  Delay/1 -> Product1/1
  DC Bus Voltage/1 -> Product3/2
  Product1/1 -> Product3/1
  Product3/1 -> ValphaBeta/1
  CosSin/1 -> Delay/1
  Gain/1 -> Abs/1

== system CRL_MCLV_V2_33EP256MC506_SlidingModeObserver_DualShunt_R2015a/DUAL SHUNT Center Aligned ==
  idx (in) : Inport
  PWM (abc) : Inport  Port=2
  MOTOR Cmd : Subsystem
  MOTOR - Board Sensor : Subsystem
  Pot [-1 1] : Outport
  Theta [0-1] : Outport  Port=2
  Iab (A) : Outport  Port=3
  DC Bus (V) : Outport  Port=4
  wires:
  idx (in)/1 -> MOTOR Cmd/1(idx in)
  MOTOR - Board Sensor/2(Iab (A)) -> Iab (A)/1
  PWM (abc)/1 -> MOTOR Cmd/2(PWM (abc))
  MOTOR - Board Sensor/4(Pot) -> Pot [-1 1]/1
  MOTOR - Board Sensor/1(DC Bus (V)) -> DC Bus (V)/1
  MOTOR Cmd/1(idx out) -> MOTOR - Board Sensor/1(idx (in))
  MOTOR - Board Sensor/3(Theta) -> Theta [0-1]/1

== system CRL_MCLV_V2_33EP256MC506_SlidingModeObserver_DualShunt_R2015a/Invert Current Sign For reversed rotation ==
  Iab : Inport
  Gain : Inport  Port=2
  Compare To Zero1 : simulink/Logic and Bit Operations/Compare To Zero  relop=>=  OutDataTypeStr=boolean
  Gain4 : Gain  Gain=-1  SaturateOnIntegerOverflow=on  OutDataTypeStr=Inherit: Same as input
  Switch3 : Switch  Criteria=u2 ~= 0  Threshold=250
  "Iab_ " : Outport
  wires:
  Gain4/1 -> Switch3/3
  Compare To Zero1/1 -> Switch3/2
  Switch3/1 -> "Iab_ "/1
  Iab/1 -> Compare To Zero1/1
  Gain/1 -> Switch3/1, Gain4/1

== system CRL_MCLV_V2_33EP256MC506_SlidingModeObserver_DualShunt_R2015a/Open Board and Motor pages ==

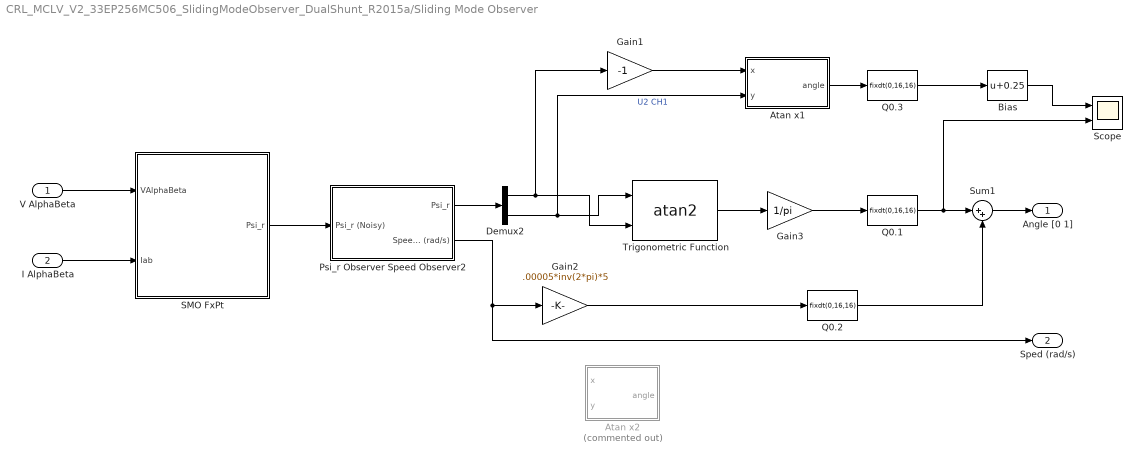
== system CRL_MCLV_V2_33EP256MC506_SlidingModeObserver_DualShunt_R2015a/Sliding Mode Observer ==
  V AlphaBeta : Inport
  I AlphaBeta : Inport  Port=2
  Atan x1 : Subsystem  AncestorBlock=Lib_MCHP_BLKDEMO_Motor/Atan x2
  Atan x2 : Subsystem  Commented=on  AncestorBlock=Lib_MCHP_BLKDEMO_Motor/Atan x2
  Bias : Bias  Bias=0.25
  Demux2 : Demux  Outputs=2
  Gain1 : Gain  Gain=-1  RndMeth=Simplest  OutDataTypeStr=Inherit: Same as input
  Gain2 : Gain  Gain=.00005*inv(2*pi)*5  OutDataTypeStr=fixdt(1,16,15)  RndMeth=Simplest
  Gain3 : Gain  Gain=1/pi  OutDataTypeStr=fixdt(1,16,15)  RndMeth=Simplest
  Psi_r Observer Speed Observer2 : Subsystem
  Q0.1 : DataTypeConversion  OutDataTypeStr=fixdt(0,16,16)  ConvertRealWorld=Stored Integer (SI)  RndMeth=Simplest
  Q0.2 : DataTypeConversion  OutDataTypeStr=fixdt(0,16,16)  RndMeth=Simplest
  Q0.3 : DataTypeConversion  OutDataTypeStr=fixdt(0,16,16)  ConvertRealWorld=Stored Integer (SI)  RndMeth=Simplest
  SMO FxPt : Subsystem
  Scope : Scope  NumInputPorts=2
      settings: YMin=-0.125~-0.12492  YMax=1.12498~1.1243
  Sum1 : Sum  Inputs=|++  OutDataTypeStr=Inherit: Same as accumulator  RndMeth=Simplest
  Trigonometric Function : Trigonometry  Operator=atan2  ApproximationMethod=CORDIC  NumberOfIterations=15
  Angle [0 1] : Outport
  Sped (rad/s) : Outport  Port=2
  wires:
  Psi_r Observer Speed Observer2/1(Psi_r) -> Demux2/1
  V AlphaBeta/1 -> SMO FxPt/1(VAlphaBeta)
  Trigonometric Function/1 -> Gain3/1
  SMO FxPt/1(Psi_r) -> Psi_r Observer Speed Observer2/1(Psi_r (Noisy))
  Psi_r Observer Speed Observer2/2(Speed we (rad/s)) -> Sped (rad/s)/1, Gain2/1
  I AlphaBeta/1 -> SMO FxPt/2(Iab)
  Sum1/1 -> Angle [0 1]/1
  Demux2/2 -> Atan x1/2(y), Trigonometric Function/1  "U2 CH1"
  Gain2/1 -> Q0.2/1
  Q0.2/1 -> Sum1/2
  Atan x1/1(angle) -> Q0.3/1
  Gain1/1 -> Atan x1/1(x)
  Q0.3/1 -> Bias/1
  Bias/1 -> Scope/1
  Q0.1/1 -> Sum1/1, Scope/2
  Demux2/1 -> Trigonometric Function/2, Gain1/1
  Gain3/1 -> Q0.1/1

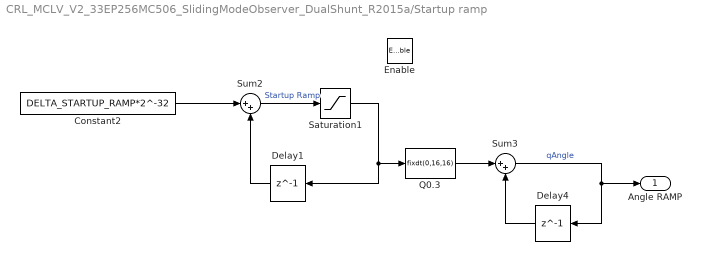
== system CRL_MCLV_V2_33EP256MC506_SlidingModeObserver_DualShunt_R2015a/Startup ramp ==
  Enable : EnablePort  StatesWhenEnabling=reset
  Constant2 : Constant  Value=DELTA_STARTUP_RAMP*2^-32  OutDataTypeStr=fixdt(0,16,32)  SampleTime=.00005
  Delay1 : Delay  DelayLength=1  InitialCondition=0
  Delay4 : Delay  DelayLength=1  InitialCondition=0
  Q0.3 : DataTypeConversion  OutDataTypeStr=fixdt(0,16,16)
  Saturation1 : Saturate  UpperLimit=DELTA_STARTUP_RAMP*2^-32*10/TS  LowerLimit=0
  Sum2 : Sum  Inputs=|++  AccumDataTypeStr=fixdt(0,32,32)  OutDataTypeStr=Inherit: Same as accumulator  RndMeth=Simplest
  Sum3 : Sum  Inputs=|++  AccumDataTypeStr=fixdt(0,16,16)  OutDataTypeStr=Inherit: Same as accumulator  RndMeth=Simplest
  Angle RAMP : Outport
  wires:
  Delay1/1 -> Sum2/2
  Saturation1/1 -> Delay1/1, Q0.3/1
  Sum2/1 -> Saturation1/1  "Startup Ramp"
  Sum3/1 -> Angle RAMP/1, Delay4/1  "qAngle"
  Q0.3/1 -> Sum3/1
  Constant2/1 -> Sum2/1
  Delay4/1 -> Sum3/2

== system CRL_MCLV_V2_33EP256MC506_SlidingModeObserver_DualShunt_R2015a/Switch from OpenLoop to Closed Loop ==
  Speed : Inport
  Delay1 : Delay  DelayLength=1  InitialCondition=[0]
  Logical Operator1 : Logic  Operator=OR  AllPortsSameDT=off  OutDataTypeStr=boolean
  Rate Transition8 : RateTransition  OutPortSampleTime=.01
  Switching Speed (rad/s Electrical) : simulink/Logic and Bit Operations/Compare To Constant  relop=>  const=250  OutDataTypeStr=boolean
  ClosedLoop 0/1 : Outport
  wires:
  Logical Operator1/1 -> Delay1/1
  Switching Speed (rad/s Electrical)/1 -> Logical Operator1/2
  Delay1/1 -> ClosedLoop 0/1/1, Logical Operator1/1
  Rate Transition8/1 -> Switching Speed (rad/s Electrical)/1
  Speed/1 -> Rate Transition8/1

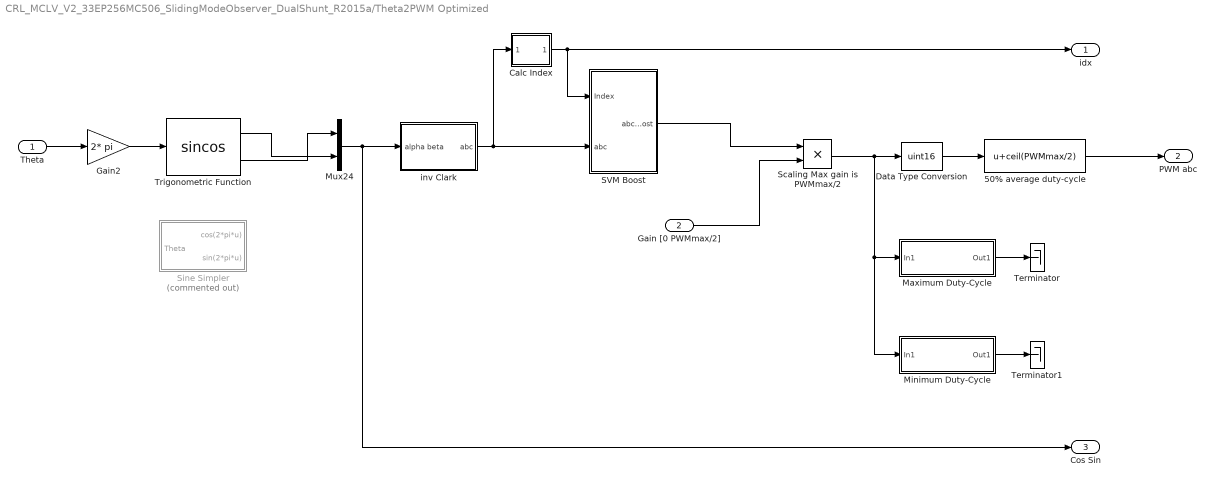
== system CRL_MCLV_V2_33EP256MC506_SlidingModeObserver_DualShunt_R2015a/Theta2PWM Optimized ==
  Theta : Inport  OutDataTypeStr=fixdt(0,16,16)
  Gain [0 PWMmax/2] : Inport  Port=2  OutMin=[-PWMmax/2]  OutMax=[PWMmax/2]
  50% average duty-cycle : Bias  Bias=ceil(PWMmax/2)
  Calc Index : Subsystem
  Data Type Conversion : DataTypeConversion  OutDataTypeStr=uint16  ConvertRealWorld=Stored Integer (SI)
  Gain2 : Gain  Gain=2* pi  OutDataTypeStr=fixdt(0,16,13)  RndMeth=Convergent
  Maximum Duty-Cycle : Subsystem
  Minimum Duty-Cycle : Subsystem
  Mux24 : Mux  Inputs=2
  SVM Boost : Subsystem
  Scaling Max gain is PWMmax/2 : Product  Inputs=**  OutDataTypeStr=int16
  Sine Simpler : Subsystem  Commented=on
  Terminator : Terminator
  Terminator1 : Terminator
  Trigonometric Function : Trigonometry  Operator=sincos  ApproximationMethod=CORDIC  NumberOfIterations=15
  inv Clark : Subsystem
  idx : Outport
  PWM abc : Outport  Port=2
  Cos Sin : Outport  Port=3
  wires:
  Mux24/1 -> inv Clark/1(alpha beta), Cos Sin/1
  Minimum Duty-Cycle/1(Out1) -> Terminator1/1
  Maximum Duty-Cycle/1(Out1) -> Terminator/1
  Scaling Max gain is PWMmax/2/1 -> Minimum Duty-Cycle/1(In1), Maximum Duty-Cycle/1(In1), Data Type Conversion/1
  Gain [0 PWMmax/2]/1 -> Scaling Max gain is PWMmax/2/2
  Calc Index/1(Idx) -> SVM Boost/1(Index), idx/1
  inv Clark/1(abc) -> Calc Index/1(In1), SVM Boost/2(abc)
  Theta/1 -> Gain2/1
  SVM Boost/1(abc boost) -> Scaling Max gain is PWMmax/2/1
  50% average duty-cycle/1 -> PWM abc/1
  Data Type Conversion/1 -> 50% average duty-cycle/1
  Trigonometric Function/2 -> Mux24/1
  Trigonometric Function/1 -> Mux24/2
  Gain2/1 -> Trigonometric Function/1

== system CRL_MCLV_V2_33EP256MC506_SlidingModeObserver_DualShunt_R2015a/reverse sign ==
  Sign : Inport
  Gain : Inport  Port=2
  Compare To Zero1 : simulink/Logic and Bit Operations/Compare To Zero  relop=>=  OutDataTypeStr=boolean
  Gain4 : Gain  Gain=-1  SaturateOnIntegerOverflow=on  OutDataTypeStr=Inherit: Same as input
  Switch3 : Switch  Criteria=u2 ~= 0  Threshold=250
  Gain_ : Outport
  wires:
  Sign/1 -> Compare To Zero1/1
  Switch3/1 -> Gain_/1
  Compare To Zero1/1 -> Switch3/2
  Gain4/1 -> Switch3/3
  Gain/1 -> Gain4/1, Switch3/1

== system CRL_MCLV_V2_33EP256MC506_SlidingModeObserver_DualShunt_R2015a/DUAL SHUNT Center Aligned/MOTOR Cmd ==
  idx in : Inport
  PWM (abc) : Inport  Port=2
  Dead time Compensation : Bias  Bias=round( (2e-6/5e-5) *PWMmax )
  Demux : Demux  Outputs=3
  PWM High Speed : MCHP_Blockset/PWM IO/PWM High Speed  pop1=[1]  chk1="[1  1  1  0]"  chkHL1="[1  1  1  1  1  1  1 ; 1  1  1  1  1  1  1]"  maxP1="[5e-05       5e-05       5e-05       0.001       0.001       0.001       0.001 ; 0.001       0.001       1e-06       0.001       0.001       0.001       0.001]"  InitP2="[5e-05       5e-05       5e-05       0.001       0.001       0.001       0.001 ; 0.001       0.001       0.001       0.001       0.001       0.001       0.001]"  chkP2="[0  0  0  1  1  1  1 ; 1  0  0  1  1  1  1]"  InitDC="[4   4   4  50  50  50  50 ; 0.001        0.001        0.001           50           50           50           50]"  chkDC="[1  1  1  1  1  1  1 ; 0  0  0  1  1  1  1]"  InitPh="[0           0           0       0.001       0.001       0.001       0.001 ; 0           0           0       0.001       0.001       0.001       0.001]"  chkPh="[0  0  0  1  1  1  1 ; 0  0  0  1  1  1  1]"  edSEvTrigx={'0','-1','-1','-1','-1','-1','-1'}  chkSEvTrigx="[0  0  0  1  1  1  1]"  popFlt="[2  2  2  1  1  1  1]"  popFltPin="[20  20  20   4   4   4   4]"  popFltPinRp="[1  1  1  1  1  1  1]"  popFltActivH="[2  2  2  1  1  1  1]"  popFltForceH="[2  2  2  2  2  2  2]"  popFltForceL="[1  1  1  1  1  1  1]"  chkFltBlkOut="[0  0  0  0  0  0  0]"  popIndepFaultMode="[1  1  1  1  1  1  1]"  popCurEnabled="[1  1  1  1  1  1  1]"  popCurPin="[33  31  32  16  16  16  16]"  popCurActiveH="[1  1  1  1  1  1  1]"  popCurForceH="[2  1  2  1  1  1  1]"  popCurForceL="[2  1  2  1  1  1  1]"  ChkCurBlkOut="[1  0  0  0  0  0  0]"  ChkCurBlkOutTime="[1  0  1  0  0  0  0]"  popBLANKSEL="[1  1  1  1  1  1  1]"  popBPHHBPHL="[1  1  1  1  1  1  1]"  popBPLHBPLL="[1  1  1  1  1  1  1]"  popFLTLEBEN_CLLEBEN="[1  1  1  1  1  1  1]"  popPHR_PHF="[2  1  1  1  1  1  1]"  popPLR_PLF="[3  1  1  1  1  1  1]"  edLEB={ '100e-9','50e-9','150e-9','50e-9','50e-9','50e-9','50e-9'}  popDT="[1  1  1  3  3  3  3]"  edDTRx="[0           0           0       1e-05       1e-05       1e-05       1e-05]"  edAltDTRx="[2e-06       2e-06       2e-06       1e-05       1e-05       1e-05       1e-05]"  S_INPUT="[5  5  5]"  S_INPUT_Size="[1  1  1]"  S_OUTPUT=[]  S_OUTPUT_Size=[]  S_DWORK_Type=[]  S_DWORK_Size=[]  ADC_VARTRIG={PWM Primary Special Event Trigger;6}  SampleTime=-1  ORDERING=None  MCHP_PORT={PWM1 Fault}{FLT32}4:0:B4;{PWM2 Fault}{FLT32}4:0:B4;{PWM3 Fault}{FLT32}4:0:B4;{PWM1H}{PWM1H}4:4:B14;{PWM1L}{PWM1L}4:4:B15;{PWM2H}{PWM2H}4:4:B12;{PWM2L}{PWM2L}4:4:B13;{PWM3H}{PWM3H}4:4:B10;{PWM3L}{PWM3L}4:4:B11;  MCHP_MASTERLINK=CRL_MCLV_V2_33EP256MC506_SlidingModeObserver_DualShunt_R2015a/Microchip Master  MCHP_VERSION=v3.38
  Saturation low side turn on errate workaround + errata for Phase shift (times 2) : Saturate  UpperLimit=PWMmax  LowerLimit=round( (2e-6/5e-5) *PWMmax )* 2
  int to uint : DataTypeConversion  OutDataTypeStr=uint16  ConvertRealWorld=Stored Integer (SI)
  idx out : Outport
  wires:
  idx in/1 -> idx out/1
  Demux/1 -> PWM High Speed/1
  Demux/3 -> PWM High Speed/3
  Demux/2 -> PWM High Speed/2
  int to uint/1 -> Saturation low side turn on errate workaround + errata for Phase shift (times 2)/1
  Saturation low side turn on errate workaround + errata for Phase shift (times 2)/1 -> Demux/1
  Dead time Compensation/1 -> int to uint/1
  PWM (abc)/1 -> Dead time Compensation/1

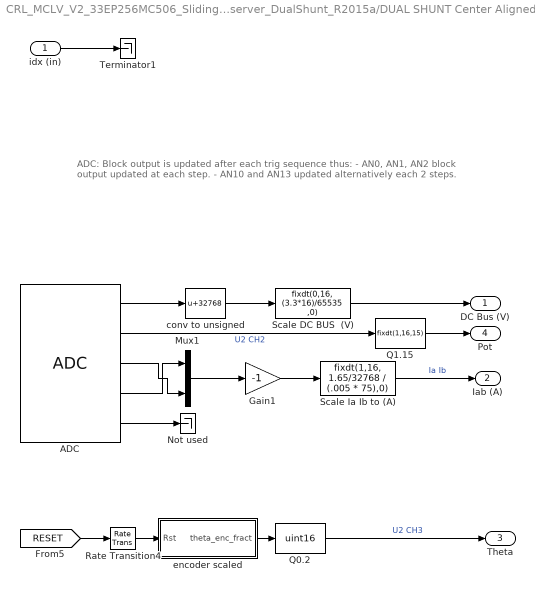
== system CRL_MCLV_V2_33EP256MC506_SlidingModeObserver_DualShunt_R2015a/DUAL SHUNT Center Aligned/MOTOR - Board Sensor ==
  note: ADC:
      | Block output is updated after each trig sequence thus:
      | - AN0, AN1, AN2 block output updated at each step.
      | - AN10 and AN13 updated alternatively each 2 steps.
  idx (in) : Inport
  ADC : MCHP_Blockset/Analog IO/ADC  Priority=5  ADC_REF=1  Mode=10 bits (allows exact simultaneous sampling)  FORM="sddd dddd dddd 0000  ==> Signed fractional"  ADC_R="< 5    kOhm"  nSAMPLECHANNELS=CH0 : CH1 : CH2 : CH3  nSAMPLECHANNELS_12bits=CH0 only  SIMULTANEOUS=Simultaneously on all Channels  ADxCSS=[10 13]  MUXA_CH0N=off  MUXA_CH123=Dynamic Options  MUXA_CH123_TXT=AN0 : AN1 : AN2  MUXB_CH0=AN1  MUXB_CH0N=on  MUXB_CH123=Dynamic Options  MUXB_CH123_TXT=AN0 : AN1 : AN2  SequenceRepeat=1  SequenceTiming=are done as fast as possible ; triggered by user define source  SSRC_SSRCG=Dynamic Options  SSRC_SSRCG_TXT=6  Update_BlockOutput=After each trig and conversion sequence  Trig_TimeStep=with each update of the ADC block output  ADC_DMA_CHANNEL=Use Interrupt instead of DMA  SampleTime=5e-05  Info=Total Time for Sample & Conversion : 8.9143e-06s including 3.4286e-07s (x 2) sample time.  MCHP_PORT={Analog Input 0}{AN0}15:2:A0;{Analog Input 1}{AN1}15:2:A1;{Analog Input 2}{AN2}15:2:B0;{Analog Input 10}{AN10}15:2:A12;{Analog Input 13}{AN13}15:2:E13;  MCHP_MASTERLINK=CRL_MCLV_V2_33EP256MC506_SlidingModeObserver_DualShunt_R2015a/Microchip Master  ADC_TIMING=[8.9142857142857144e-06]
  Gain1 : Gain  Gain=-1  SaturateOnIntegerOverflow=on  OutDataTypeStr=Inherit: Same as input
  Mux1 : Mux  Inputs=2
  Not used : Terminator
  Q0.2 : DataTypeConversion  OutDataTypeStr=uint16  ConvertRealWorld=Stored Integer (SI)
  Q1.15 : DataTypeConversion  OutDataTypeStr=fixdt(1,16,15)  ConvertRealWorld=Stored Integer (SI)
  Rate Transition4 : RateTransition  X0=1
  Scale DC BUS  (V) : DataTypeConversion  OutDataTypeStr=fixdt(0,16, (3.3*16)/65535 ,0)  ConvertRealWorld=Stored Integer (SI)
  Scale Ia Ib to (A) : DataTypeConversion  OutDataTypeStr=fixdt(1,16, 1.65/32768 / (.005 * 75),0)  ConvertRealWorld=Stored Integer (SI)
  Terminator1 : Terminator
  conv to unsigned : Bias  Bias=32768
  encoder scaled : Subsystem
  DC Bus (V) : Outport
  Iab (A) : Outport  Port=2
  Theta : Outport  Port=3
  Pot : Outport  Port=4
  wires:
  Q1.15/1 -> Pot/1
  idx (in)/1 -> Terminator1/1
  Scale DC BUS  (V)/1 -> DC Bus (V)/1
  Scale Ia Ib to (A)/1 -> Iab (A)/1  "Ia Ib"
  Q0.2/1 -> Theta/1  "U2 CH3"
  ADC/2 -> Q1.15/1  "U2 CH2"
  [RESET] -> Rate Transition4/1
  encoder scaled/1(theta_enc_fract) -> Q0.2/1
  ADC/3 -> Mux1/2
  ADC/4 -> Mux1/1
  conv to unsigned/1 -> Scale DC BUS  (V)/1
  Mux1/1 -> Gain1/1
  ADC/1 -> conv to unsigned/1
  Rate Transition4/1 -> encoder scaled/1(Rst)
  ADC/5 -> Not used/1
  Gain1/1 -> Scale Ia Ib to (A)/1
